simulink model "Batbot_SIM"  (Simulink 7.5)
settings: Solver=ode45  StartTime=0.0  StopTime=5  FixedStep=0.1  RelTol=1e-3
values from neighbouring files (symbols this model uses):
  F_flapping = 1000    [SimulationFB.m]
  step_2 = tf/(col-1)    [SimulationFB.m]    (also in inverse_kinematicsFULLFB.m = 0.0114285714286)
libraries: mblibv1 x76, motdrv_lib x8, simulink x7
(part 1 of 3)
settings Model: Creator=Administrador  LastModifiedBy=Administrador
settings SimMechanicsCC: VisOnUpdateDiagram=on  VisDuringSimulation=on  LastVizWinPosition=[75 76 659 717]  CamPosition=[-6.19696;5.48902;7.70944;]  CamTarget=[-0.0161827;-0.0229426;0.00388461;]  CamUpVector=[0.159937;0.859072;-0.486225;]  CamHeight=0.433034  VisBackgroundColor=[1;1;1;]  DefaultBodyColor=[1;0;0;]

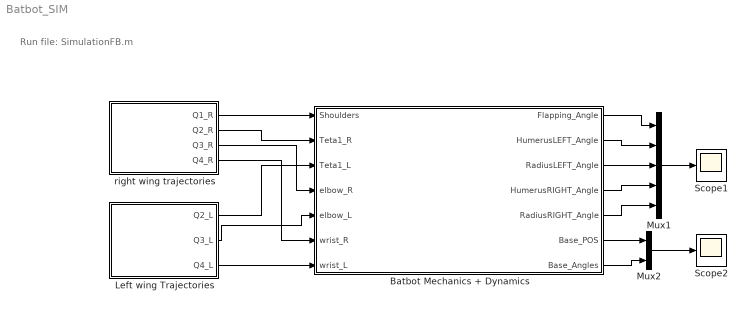
== system Batbot_SIM ==
  note: Run file: SimulationFB.m
  Batbot Mechanics + Dynamics : Subsystem
      mask Display: image(imread('batbot.jpg'))
  "Left wing Trajectories " : Subsystem
  Mux1 : Mux  Inputs=5
  Mux2 : Mux  Inputs=2
  Scope1 : Scope
  Scope2 : Scope
      settings: SaveName=ScopeData2
  right wing trajectories : Subsystem
  wires:
  right wing trajectories/1(Q1_R) -> Batbot Mechanics + Dynamics/1(Shoulders)
  right wing trajectories/2(Q2_R) -> Batbot Mechanics + Dynamics/2(Teta1_R)
  "Left wing Trajectories "/1(Q2_L) -> Batbot Mechanics + Dynamics/3(Teta1_L)
  right wing trajectories/3(Q3_R) -> Batbot Mechanics + Dynamics/4(elbow_R)
  "Left wing Trajectories "/2(Q3_L) -> Batbot Mechanics + Dynamics/5(elbow_L)
  "Left wing Trajectories "/3(Q4_L) -> Batbot Mechanics + Dynamics/7(wrist_L)
  right wing trajectories/4(Q4_R) -> Batbot Mechanics + Dynamics/6(wrist_R)
  Batbot Mechanics + Dynamics/1(Flapping_Angle) -> Mux1/1
  Batbot Mechanics + Dynamics/2(HumerusLEFT_Angle) -> Mux1/2
  Batbot Mechanics + Dynamics/3(RadiusLEFT_Angle) -> Mux1/3
  Batbot Mechanics + Dynamics/4(HumerusRIGHT_Angle) -> Mux1/4
  Mux1/1 -> Scope1/1
  Batbot Mechanics + Dynamics/5(RadiusRIGHT_Angle) -> Mux1/5
  Batbot Mechanics + Dynamics/6(Base_POS) -> Mux2/1
  Batbot Mechanics + Dynamics/7(Base_Angles) -> Mux2/2
  Mux2/1 -> Scope2/1
